simulink model "sampleModel1968"  (R2023a)
settings: Solver=VariableStepAuto  StartTime=0.0  StopTime=10.0  RelTol=1e-3
libraries: hdlsllib x8, simulink x5
settings Model: Creator=user1  LastModifiedBy=user1

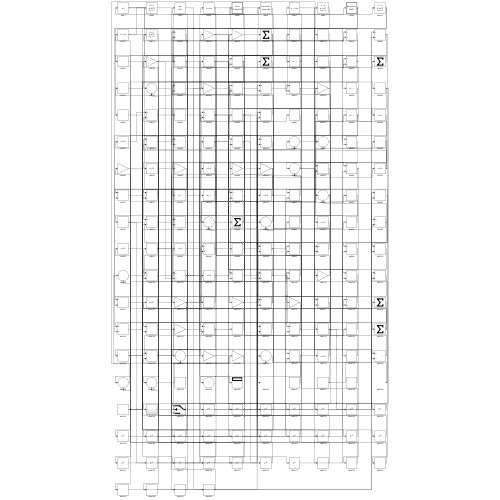
[thumbnail: Simulink's stored preview of the top-level diagram]
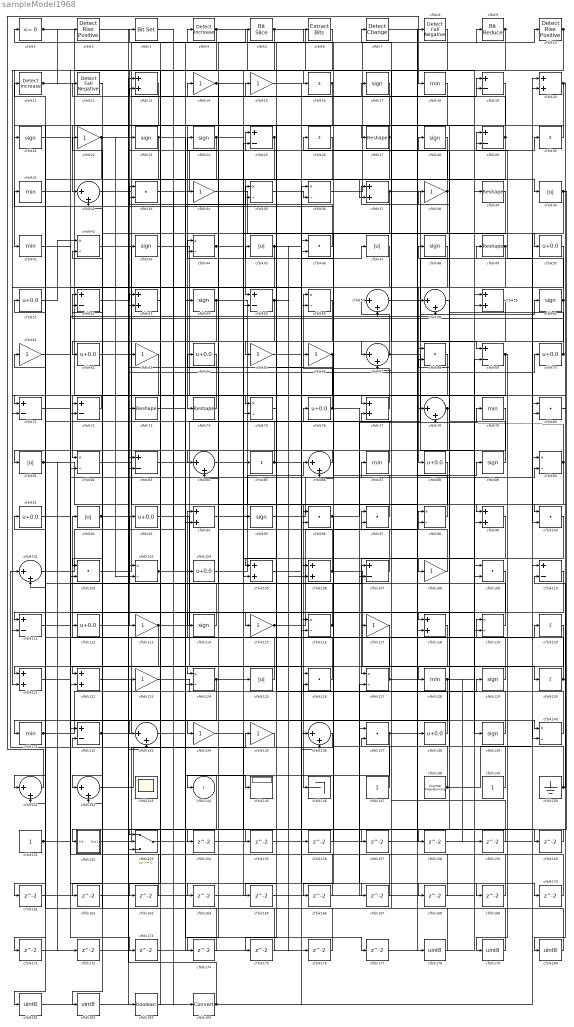
== system sampleModel1968 ==
  cfblk1 : hdlsllib/Logic and Bit Operations/Compare To Zero  relop=<=  OutDataTypeStr=boolean
  cfblk10 : hdlsllib/Logic and Bit Operations/Detect Rise Positive  vinit=0  OutDataTypeStr=boolean
  cfblk{33,46,68,80,96..97,100,102,109,126,137} (11 alike) : DotProduct  OutDataTypeStr=Inherit: Inherit via internal rule
  cfblk{32,57..58,67,78,84,86,101,133,136,141..142} (12 alike) : Sum  Inputs=|++
  cfblk{35..36,42,44,56,75,82,90,98,103,116,119,124,127,140} (15 alike) : Product  Inputs=*/  RndMeth=Zero  SaturateOnIntegerOverflow=on
  cfblk{50..51,62,64,70,76,88,91,93,104,112,138} (12 alike) : Bias  Bias=0.0  SaturateOnIntegerOverflow=off
  cfblk{13,20,37,53,59,77,94,99,105..106,118,121..122} (13 alike) : Sum
  cfblk{19,25,29,52,55,69,71..72,83,107,110..111,132} (13 alike) : Sum  Inputs=+-
  cfblk{14..15,22,34,38,61,63,65..66,108,113,115,117,123,134..135} (16 alike) : Gain
  cfblk11 : simulink/Logic and Bit Operations/Detect Increase  vinit=0.0  OutDataTypeStr=boolean
      settings: LibrarySourceBlock=|
      | hdlsllib/Logic and Bit
      | Operations/Detect
      | Increase
  cfblk{17,21,23..24,28,43,48,54,60,89,95,114,129,139} (14 alike) : Signum
  cfblk12 : hdlsllib/Logic and Bit Operations/Detect Fall Negative  vinit=0  OutDataTypeStr=boolean
  cfblk{16,26,30,85,120,130} (6 alike) : Sum  Inputs=+
  cfblk{40,45,47,81,92,125} (6 alike) : Abs  SaturateOnIntegerOverflow=off
  cfblk{18,31,41,79,87,128,131} (7 alike) : MinMax
  cfblk143 : Scope
      settings: Floating=on
  cfblk145 : Display
  cfblk146 : Terminator
  cfblk147 : Constant  SampleTime=-1
  cfblk148 : hdlsllib/Sources/Counter Free-Running  NumBits=16  tsamp=-1
  cfblk149 : Constant  SampleTime=-1
  cfblk150 : Ground
  cfblk151 : Constant  SampleTime=-1
  cfblk152 : Subsystem
      settings: LibrarySourceBlock=|
      | hdlsllib/Ports &
      | Subsystems/Subsystem
  cfblk153 : Switch  SaturateOnIntegerOverflow=off  InputSameDT=off
  cfblk{154..177} (24 alike) : Delay  SampleTime=1
  cfblk{178..182} (5 alike) : DataTypeConversion  OutDataTypeStr=uint8  SaturateOnIntegerOverflow=off  RndMeth=Floor
  cfblk183 : DataTypeConversion  OutDataTypeStr=boolean  SaturateOnIntegerOverflow=off  RndMeth=Floor
  cfblk184 : DataTypeConversion  SaturateOnIntegerOverflow=off  RndMeth=Floor
  cfblk2 : hdlsllib/Logic and Bit Operations/Detect Rise Positive  vinit=0  OutDataTypeStr=boolean
  cfblk{27,39,49,73..74} (5 alike) : Reshape
  cfblk3 : simulink/Logic and Bit Operations/Bit Set  iBit=0
      settings: LibrarySourceBlock=|
      | hdlsllib/Logic and Bit
      | Operations/Bit Set
  cfblk4 : simulink/Logic and Bit Operations/Detect Increase  vinit=0.0  OutDataTypeStr=boolean
      settings: LibrarySourceBlock=|
      | hdlsllib/Logic and Bit
      | Operations/Detect
      | Increase
  cfblk5 : hdlsllib/Logic and Bit Operations/Bit Slice  lidx=7  ridx=0
  cfblk6 : simulink/Logic and Bit Operations/Extract Bits  bitsToExtract=Upper half  numBits=8  bitIdxRange=[0 7]  outScalingMode=Preserve fixed-point scaling
      settings: LibrarySourceBlock=|
      | hdlsllib/Logic and Bit
      | Operations/Extract Bits
  cfblk7 : simulink/Logic and Bit Operations/Detect Change  vinit=0  OutDataTypeStr=boolean
      settings: LibrarySourceBlock=|
      | hdlsllib/Logic and Bit
      | Operations/Detect
      | Change
  cfblk8 : hdlsllib/Logic and Bit Operations/Detect Fall Negative  vinit=0  OutDataTypeStr=boolean
  cfblk9 : hdlsllib/Logic and Bit Operations/Bit Reduce  mode=AND
  cfblk144 : Outport  VectorParamsAs1DForOutWhenUnconnected=off
  wires:
  cfblk32/1 -> cfblk40/1
  cfblk103/1 -> cfblk76/1, cfblk34/1, cfblk6/1
  cfblk137/1 -> cfblk89/1, cfblk154/1
  cfblk117/1 -> cfblk121/1
  cfblk131/1 -> cfblk97/1, cfblk141/2, cfblk173/1
  cfblk1/1 -> cfblk99/1, cfblk78/1
  cfblk19/1 -> cfblk74/1
  cfblk136/1 -> cfblk101/1
  cfblk50/1 -> cfblk88/1
  cfblk141/1 -> cfblk18/1
  cfblk147/1 -> cfblk15/1
  cfblk78/1 -> cfblk108/1, cfblk102/1
  cfblk6/1 -> cfblk41/1
  cfblk120/1 -> cfblk122/1
  cfblk68/1 -> cfblk77/1
  cfblk28/1 -> cfblk55/1
  cfblk118/1 -> cfblk131/1
  cfblk36/1 -> cfblk10/1
  cfblk13/1 -> cfblk32/1
  cfblk104/1 -> cfblk86/1
  cfblk96/1 -> cfblk79/1, cfblk166/1
  cfblk51/1 -> cfblk42/1
  cfblk76/1 -> cfblk45/1, cfblk169/1
  cfblk116/1 -> cfblk24/1, cfblk104/1
  cfblk122/1 -> cfblk134/1
  cfblk82/1 -> cfblk9/1
  cfblk94/1 -> cfblk95/1
  cfblk102/1 -> cfblk19/1
  cfblk130/1 -> cfblk17/1, cfblk97/2
  cfblk9/1 -> cfblk113/1, cfblk121/2
  cfblk33/1 -> cfblk25/1
  cfblk99/1 -> cfblk127/1
  cfblk4/1 -> cfblk16/1, cfblk73/1
  cfblk30/1 -> cfblk21/1
  cfblk54/1 -> cfblk138/1, cfblk107/2, cfblk182/1
  cfblk22/1 -> cfblk27/1, cfblk103/2, cfblk82/2
  cfblk34/1 -> cfblk109/1
  cfblk95/1 -> cfblk90/2
  cfblk16/1 -> cfblk75/1, cfblk141/1
  cfblk106/1 -> cfblk130/1, cfblk44/2
  cfblk113/1 -> cfblk49/1, cfblk153/2, cfblk35/2
  cfblk121/1 -> cfblk124/1
  cfblk124/1 -> cfblk75/2, cfblk153/3
  cfblk123/1 -> cfblk129/1
  cfblk23/1 -> cfblk145/1, cfblk53/2
  cfblk59/1 -> cfblk65/1
  cfblk109/1 -> cfblk111/1
  cfblk39/1 -> cfblk62/1
  cfblk24/1 -> cfblk85/1, cfblk29/2, cfblk171/1
  cfblk93/1 -> cfblk146/1
  cfblk37/1 -> cfblk69/1, cfblk105/1
  cfblk139/1 -> cfblk48/1
  cfblk129/1 -> cfblk92/1
  cfblk110/1 -> cfblk117/1
  cfblk90/1 -> cfblk144/1, cfblk78/2
  cfblk67/1 -> cfblk139/1, cfblk57/1, cfblk119/2
  cfblk56/1 -> cfblk124/2
  cfblk77/1 -> cfblk56/1
  cfblk115/1 -> cfblk98/1, cfblk35/1
  cfblk91/1 -> cfblk87/1
  cfblk119/1 -> cfblk93/1
  cfblk61/1 -> cfblk140/1
  cfblk49/1 -> cfblk111/2, cfblk59/2
  cfblk98/1 -> cfblk44/1
  cfblk128/1 -> cfblk120/1, cfblk159/1, cfblk161/1
  cfblk132/1 -> cfblk94/1, cfblk133/2
  cfblk12/1 -> cfblk142/1
  cfblk100/1 -> cfblk128/1
  cfblk40/1 -> cfblk152/1(In1), cfblk100/2
  cfblk125/1 -> cfblk22/1
  cfblk81/1 -> cfblk123/1, cfblk172/1
  cfblk43/1 -> cfblk136/2
  cfblk11/1 -> cfblk59/1, cfblk2/1
  cfblk148/1 -> cfblk110/1, cfblk1/1
  cfblk114/1 -> cfblk61/1
  cfblk72/1 -> cfblk71/1
  cfblk83/1 -> cfblk60/1
  cfblk70/1 -> cfblk26/1, cfblk52/1
  cfblk138/1 -> cfblk5/1
  cfblk112/1 -> cfblk66/1
  cfblk88/1 -> cfblk126/1
  cfblk69/1 -> cfblk96/2, cfblk179/1
  cfblk152/1(Out1) -> cfblk135/1
  cfblk87/1 -> cfblk51/1
  cfblk85/1 -> cfblk64/1, cfblk58/2
  cfblk45/1 -> cfblk122/2, cfblk106/2, cfblk168/1
  cfblk108/1 -> cfblk14/1
  cfblk14/1 -> cfblk50/1, cfblk37/2, cfblk84/2
  cfblk127/1 -> cfblk33/1, cfblk140/2
  cfblk38/1 -> cfblk28/1, cfblk86/2
  cfblk149/1 -> cfblk38/1
  cfblk142/1 -> cfblk125/1
  cfblk5/1 -> cfblk39/1, cfblk105/2
  cfblk84/1 -> cfblk55/2
  cfblk63/1 -> cfblk71/2
  cfblk27/1 -> cfblk23/1, cfblk162/1
  cfblk60/1 -> cfblk68/1, cfblk29/1, cfblk116/2
  cfblk29/1 -> cfblk12/1, cfblk102/2
  cfblk140/1 -> cfblk68/2
  cfblk35/1 -> cfblk36/2
  cfblk89/1 -> cfblk37/1
  cfblk31/1 -> cfblk56/2
  cfblk8/1 -> cfblk67/1
  cfblk10/1 -> cfblk98/2, cfblk72/2
  cfblk42/1 -> cfblk137/1
  cfblk153/1 -> cfblk8/1
  cfblk52/1 -> cfblk53/1
  cfblk86/1 -> cfblk81/1
  cfblk105/1 -> cfblk47/1
  cfblk133/1 -> cfblk19/2
  cfblk151/1 -> cfblk107/1, cfblk57/2, cfblk119/1
  cfblk64/1 -> cfblk82/1
  cfblk107/1 -> cfblk4/1
  cfblk57/1 -> cfblk20/2
  cfblk18/1 -> cfblk63/1
  cfblk55/1 -> cfblk133/1, cfblk176/1
  cfblk3/1 -> cfblk184/1
  cfblk15/1 -> cfblk118/1
  cfblk126/1 -> cfblk91/1
  cfblk21/1 -> cfblk118/2
  cfblk25/1 -> cfblk43/1, cfblk84/1
  cfblk66/1 -> cfblk114/1, cfblk83/2
  cfblk46/1 -> cfblk13/2
  cfblk20/1 -> cfblk58/1, cfblk100/1
  cfblk74/1 -> cfblk72/1
  cfblk92/1 -> cfblk30/1, cfblk70/1, cfblk52/2
  cfblk44/1 -> cfblk109/2, cfblk96/1
  cfblk97/1 -> cfblk31/1
  cfblk101/1 -> cfblk54/1
  cfblk135/1 -> cfblk132/2
  cfblk150/1 -> cfblk137/2, cfblk110/2
  cfblk17/1 -> cfblk115/1
  cfblk154/1 -> cfblk90/1
  cfblk75/1 -> cfblk155/1
  cfblk155/1 -> cfblk46/1
  cfblk65/1 -> cfblk156/1
  cfblk156/1 -> cfblk126/2
  cfblk2/1 -> cfblk157/1
  cfblk157/1 -> cfblk67/2
  cfblk58/1 -> cfblk158/1
  cfblk158/1 -> cfblk20/1
  cfblk159/1 -> cfblk77/2
  cfblk134/1 -> cfblk160/1
  cfblk160/1 -> cfblk153/1
  cfblk161/1 -> cfblk127/2
  cfblk162/1 -> cfblk25/2
  cfblk53/1 -> cfblk163/1
  cfblk163/1 -> cfblk132/1
  cfblk111/1 -> cfblk164/1
  cfblk164/1 -> cfblk69/2
  cfblk79/1 -> cfblk165/1
  cfblk165/1 -> cfblk106/1
  cfblk166/1 -> cfblk103/1
  cfblk71/1 -> cfblk167/1
  cfblk167/1 -> cfblk36/1
  cfblk168/1 -> cfblk32/2
  cfblk169/1 -> cfblk33/2
  cfblk41/1 -> cfblk170/1
  cfblk170/1 -> cfblk142/2
  cfblk171/1 -> cfblk94/2
  cfblk172/1 -> cfblk136/1
  cfblk173/1 -> cfblk116/1
  cfblk26/1 -> cfblk174/1
  cfblk174/1 -> cfblk13/1
  cfblk47/1 -> cfblk175/1
  cfblk175/1 -> cfblk42/2
  cfblk176/1 -> cfblk101/2
  cfblk73/1 -> cfblk177/1
  cfblk177/1 -> cfblk99/2
  cfblk7/1 -> cfblk178/1
  cfblk178/1 -> cfblk112/1
  cfblk179/1 -> cfblk7/1
  cfblk80/1 -> cfblk180/1
  cfblk180/1 -> cfblk11/1
  cfblk48/1 -> cfblk181/1
  cfblk181/1 -> cfblk80/1
  cfblk182/1 -> cfblk80/2
  cfblk62/1 -> cfblk183/1
  cfblk183/1 -> cfblk3/1
  cfblk184/1 -> cfblk83/1, cfblk46/2

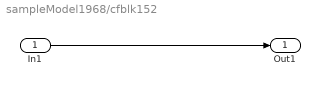
== system sampleModel1968/cfblk152 ==
  In1 : Inport
  Out1 : Outport
  wires:
  In1/1 -> Out1/1
